simulink model "UAV_Research_Environment"  (R2025a)
settings: Solver=ode23t  StartTime=0.0  StopTime=130  MaxStep=2e-3  RelTol=1e-4  AbsTol=1e-3  EnableMultiTasking=on
InitFcn:
  | skipInitialization = false;
  | 
  | if evalin('base', ...
  |         'exist(''CONTROLLER_TUNING_ACTIVE'',''var'')')
  | 
  |     skipInitialization = evalin('base', ...
  |         'logical(CONTROLLER_TUNING_ACTIVE)');
  | end
  | 
  | if ~skipInitialization
  | 
  |     icraControllerPrepared = false;
  | 
  |     hasICRAVariables = evalin('base', ...
  |         ['exist(''AUTOPILOT'',''var'') && ' ...
  |          'exist(''ICRA_ACTIVE_CONTROLLER'',''var'') && ' ...
  |          'exist(''ICRA_ACTIVE_RUN_ID'',''var'')']);
  | 
  |     if hasICRAVariables
  | 
  |         icraControllerPrepared = evalin('base', ...
  |             ['isstruct(AUTOPILOT) && ' ...
  |              'isfield(AUTOPILOT,''info'') && ' ...
  |              'isfield(AUTOPILOT.info,''ICRAControllerID'') && ' ...
  |              'strcmp(string(AUTOPILOT.info.ICRAControllerID), ' ...
  |                     'string(ICRA_ACTIVE_CONTROLLER))']);
  | 
  |     end
  | 
  |     if icraControllerPrepared
  |         skipInitialization = true;
  |     end
  | end
  | 
  | if ~skipInitialization
  | 
  |     mdl = bdroot;
  | 
  |     mdl_file = get_param(mdl, 'FileName');
  | 
  |     project_root = fileparts(mdl_file);
  | 
  |     init_file = fullfile(project_root, 'initialize_project.m');
  | 
  |     if exist(init_file, 'file')
  | 
  |         run(init_file);
  | 
  |     else
  | 
  |         error('initialize_project.m was not found in the model folder.');
  | 
  |     end
  | end
values from neighbouring files (symbols this model uses):
  A_UAV = struct()    [UAV_analytical.m]
  AUTOPILOT = struct()    [UAV_autopilot.m]
  B_UAV = struct()    [UAV_block.m]
  D = A_UAV.source.propeller_diameter_m    [UAV_analytical.m]    (also in plot_controller_results.m = permute(                  D,                  order); plot_estimator_results.m = permute(              D,              order); plot_mission_results.m = permute(                  D,                  order); plot_touchdown_diagnostics.m = permute(                  D,                  order))
  OPERATOR_MODE = OPERATOR_MODE_MANUAL    [initialize_project.m]    (also in uav_remote_gui.m = uint8(0))
  P_ENV = struct()    [Environment.m]
  P_UAV = struct()    [UAV_simscape.m]
  s = sin(angle)    [uav_remote_gui.m]
  SENSOR = struct()    [UAV_sensors.m]
  TRAJECTORY_CONFIG = struct()    [UAV_trajectories.m]
  TRAJECTORY_ID = uint8(          trajectoryIDNumeric)    [UAV_trajectories.m]
  X = reshape(                  D,                  nt,                  [])    [plot_controller_results.m]    (also in plot_estimator_results.m = reshape(              D,              nt,              []); plot_mission_results.m; plot_touchdown_diagnostics.m; plot_trajectory_3d.m)
  Y = absolutePlanNED(1,:)    [plot_trajectory_3d.m]    (also in uav_remote_gui.m = positionNED(:,1))
  Z = landedCGDown -          absolutePlanNED(3,:)    [plot_trajectory_3d.m]    (also in uav_remote_gui.m = landedCGDown-positionNED(:,3))
undefined symbols (not defined in the file or in its folder): Acceleration_ref, F, fractalcoef, Light, MIL, Position_ref, Velocity_ref, Yaw_ref, YawRate_ref
libraries: sm_lib x49, nesl_utility x29, fl_lib x17, slpidlib x16, simulink x14, ee_lib x5, sdl_lib x4, aerolibwind2 x3, aerolibatmos2 x2, sensorbarometerlib x1, sensorgpslib x1, mspsensorlib x1
(part 3 of 9)

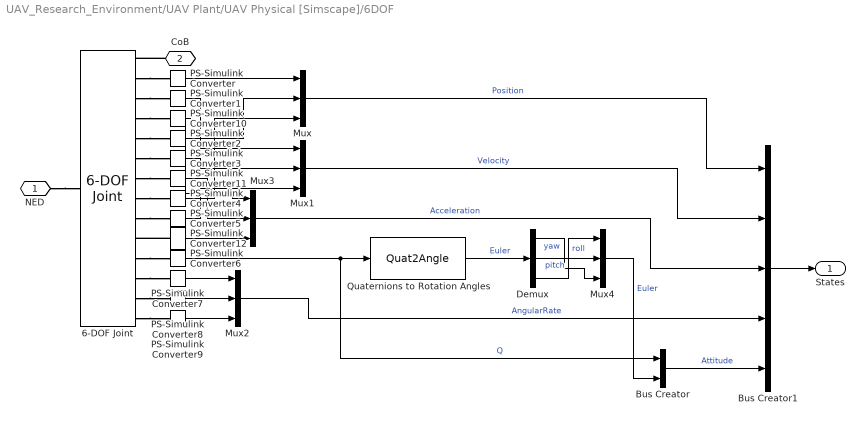
== system UAV_Research_Environment/UAV Plant/UAV Physical [Simscape]/6DOF ==
  6-DOF Joint : sm_lib/Joints/6-DOF Joint  JointMode=Normal  CompositeWrenchDir=FollowerOnBase  CompositeWrenchFrame=BaseFrame  SenseConstraintForce=off  SenseConstraintTorque=off  SenseTotalForce=off  SenseTotalTorque=off  PxPositionTargetSpecify=off  PxPositionTargetPriority=High  PxPositionTargetValue=0  PxPositionTargetValueUnits=m  PxVelocityTargetSpecify=off  PxVelocityTargetPriority=High  PxVelocityTargetValue=0  PxVelocityTargetValueUnits=m/s  PxEquilibriumPosition=0  PxEquilibriumPositionUnits=m  PxSpringStiffness=0  PxSpringStiffnessUnits=N/m  PxDampingCoefficient=0  PxDampingCoefficientUnits=N/(m/s)  PxLowerLimitSpecify=off  PxLowerLimitBound=-1  PxLowerLimitBoundUnits=m  PxLowerLimitStiffness=1e6  PxLowerLimitStiffnessUnits=N/m  PxLowerLimitDamping=1e3  PxLowerLimitDampingUnits=N/(m/s)  PxLowerLimitTransitionRegionWidth=1e-4  PxLowerLimitTransitionRegionWidthUnits=m  PxUpperLimitSpecify=off  PxUpperLimitBound=1  PxUpperLimitBoundUnits=m  PxUpperLimitStiffness=1e6  PxUpperLimitStiffnessUnits=N/m  PxUpperLimitDamping=1e3  PxUpperLimitDampingUnits=N/(m/s)  PxUpperLimitTransitionRegionWidth=1e-4  PxUpperLimitTransitionRegionWidthUnits=m  PxTorqueActuationMode=NoTorque  PxMotionActuationMode=ComputedMotion  PxSensePosition=on  PxSenseVelocity=on  PxSenseAcceleration=on  PxSenseTorqueForce=off  PxSenseLowerLimitTorqueForce=off  PxSenseUpperLimitTorqueForce=off  PyPositionTargetSpecify=off  PyPositionTargetPriority=High  PyPositionTargetValue=0  PyPositionTargetValueUnits=m  PyVelocityTargetSpecify=off  PyVelocityTargetPriority=High  PyVelocityTargetValue=0  PyVelocityTargetValueUnits=m/s  PyEquilibriumPosition=0  PyEquilibriumPositionUnits=m  PySpringStiffness=0  PySpringStiffnessUnits=N/m  PyDampingCoefficient=0  PyDampingCoefficientUnits=N/(m/s)  PyLowerLimitSpecify=off  PyLowerLimitBound=-1  PyLowerLimitBoundUnits=m  PyLowerLimitStiffness=1e6  PyLowerLimitStiffnessUnits=N/m  PyLowerLimitDamping=1e3  PyLowerLimitDampingUnits=N/(m/s)  PyLowerLimitTransitionRegionWidth=1e-4  PyLowerLimitTransitionRegionWidthUnits=m  PyUpperLimitSpecify=off  PyUpperLimitBound=1  PyUpperLimitBoundUnits=m  PyUpperLimitStiffness=1e6  PyUpperLimitStiffnessUnits=N/m  PyUpperLimitDamping=1e3  PyUpperLimitDampingUnits=N/(m/s)  PyUpperLimitTransitionRegionWidth=1e-4  PyUpperLimitTransitionRegionWidthUnits=m  PyTorqueActuationMode=NoTorque  PyMotionActuationMode=ComputedMotion  PySensePosition=on  PySenseVelocity=on  PySenseAcceleration=on  PySenseTorqueForce=off  PySenseLowerLimitTorqueForce=off  PySenseUpperLimitTorqueForce=off  PzPositionTargetSpecify=on  PzPositionTargetPriority=High  PzPositionTargetValue=P_UAV.initial_conditions.position_ned_m(3)  PzPositionTargetValueUnits=m  PzVelocityTargetSpecify=off  PzVelocityTargetPriority=High  PzVelocityTargetValue=0  PzVelocityTargetValueUnits=m/s  PzEquilibriumPosition=0  PzEquilibriumPositionUnits=m  PzSpringStiffness=0  PzSpringStiffnessUnits=N/m  PzDampingCoefficient=0  PzDampingCoefficientUnits=N/(m/s)  PzLowerLimitSpecify=off  PzLowerLimitBound=-1  PzLowerLimitBoundUnits=m  PzLowerLimitStiffness=1e6  PzLowerLimitStiffnessUnits=N/m  PzLowerLimitDamping=1e3  PzLowerLimitDampingUnits=N/(m/s)  PzLowerLimitTransitionRegionWidth=1e-4  PzLowerLimitTransitionRegionWidthUnits=m  PzUpperLimitSpecify=off  PzUpperLimitBound=1  PzUpperLimitBoundUnits=m  PzUpperLimitStiffness=1e6  PzUpperLimitStiffnessUnits=N/m  PzUpperLimitDamping=1e3  PzUpperLimitDampingUnits=N/(m/s)  PzUpperLimitTransitionRegionWidth=1e-4  PzUpperLimitTransitionRegionWidthUnits=m  PzTorqueActuationMode=NoTorque  PzMotionActuationMode=ComputedMotion  PzSensePosition=on  PzSenseVelocity=on  PzSenseAcceleration=on  PzSenseTorqueForce=off  PzSenseLowerLimitTorqueForce=off  PzSenseUpperLimitTorqueForce=off  SphPositionTargetSpecify=off  SphPositionTargetPriority=High  SphPositionTargetRotationMethod=None  SphPositionTargetFollAlignAxisA=+X  SphPositionTargetBaseAlignAxisA=+Y  SphPositionTargetFollAlignAxisB=+Y  SphPositionTargetBaseAlignAxisB=+Z  SphPositionTargetRotationStandardAxis=+Z  SphPositionTargetRotationAngle=0  SphPositionTargetRotationAngleUnits=deg  SphPositionTargetRotationArbitraryAxis=[0 0 1]  SphPositionTargetRotationSequenceAxes=FollowerAxes  SphPositionTargetRotationSequence=XYX  SphPositionTargetRotationSequenceAngles=[0 0 0]  SphPositionTargetRotationSequenceAnglesUnits=deg  SphPositionTargetRotationMatrix=[1 0 0;0 1 0;0 0 1]  SphPositionTargetQuaternion=[1 0 0 0]  SphVelocityTargetSpecify=off  SphVelocityTargetPriority=High  SphVelocityTargetValue=[0 0 0]  SphVelocityTargetValueUnits=deg/s  SphVelocityTargetInFollowerFrame=on  SphEqPosRotationMethod=None  SphEqPosFollAlignAxisA=+X  SphEqPosBaseAlignAxisA=+Y  SphEqPosFollAlignAxisB=+Y  SphEqPosBaseAlignAxisB=+Z  SphEqPosRotationStandardAxis=+Z  SphEqPosRotationAngle=0  SphEqPosRotationAngleUnits=deg  SphEqPosRotationArbitraryAxis=[0 0 1]  SphEqPosRotationSequenceAxes=FollowerAxes  SphEqPosRotationSequence=XYX  SphEqPosRotationSequenceAngles=[0 0 0]  SphEqPosRotationSequenceAnglesUnits=deg  SphEqPosRotationMatrix=[1 0 0;0 1 0;0 0 1]  SphEqPosQuaternion=[1 0 0 0]  SphSpringStiffness=0  SphSpringStiffnessUnits=N*m/deg  SphDampingCoefficient=0  SphDampingCoefficientUnits=N*m/(deg/s)  SphLowerLimitSpecify=off  SphLowerLimitBound=15  SphLowerLimitBoundUnits=deg  SphLowerLimitStiffness=1e4  SphLowerLimitStiffnessUnits=N*m/deg  SphLowerLimitDamping=10  SphLowerLimitDampingUnits=N*m/(deg/s)  SphLowerLimitTransitionRegionWidth=0.1  SphLowerLimitTransitionRegionWidthUnits=deg  SphUpperLimitSpecify=off  SphUpperLimitBound=45  SphUpperLimitBoundUnits=deg  SphUpperLimitStiffness=1e4  SphUpperLimitStiffnessUnits=N*m/deg  SphUpperLimitDamping=10  SphUpperLimitDampingUnits=N*m/(deg/s)  SphUpperLimitTransitionRegionWidth=0.1  SphUpperLimitTransitionRegionWidthUnits=deg  SphTorqueActuationMode=NoTorque  SphActuateTorqueX=off  SphActuateTorqueY=off  SphActuateTorqueZ=off  SphActuateTorque=off  SphActuationFrame=BaseFrame  SphSensePosition=on  SphSenseVelocityX=on  SphSenseVelocityY=on  SphSenseVelocityZ=on  SphSenseVelocity=off  SphSenseAccelerationX=off  SphSenseAccelerationY=off  SphSenseAccelerationZ=off  SphSenseAcceleration=off  SphSenseLowerLimitTorqueMag=off  SphSenseUpperLimitTorqueMag=off  SphSensingFrame=FollowerFrame
  Bus Creator : BusCreator  Inputs=2
  Bus Creator1 : BusCreator  Inputs=5
  Demux : Demux  Outputs=3
  Mux{,1..4} (5 alike) : Mux  Inputs=3
  PS-Simulink Converter{,1..12} (13 alike) : nesl_utility/PS-Simulink Converter  PhysicalDomain=network_engine_domain  SubClassName=ps_output  LeftPortType=input  RightPortType=output  PseudoPeriodic=off  Frequencies=[]  VectorFormat=inherit  Unit=inherit  AffineConversion=off
  Quaternions to Rotation Angles : Quat2Angle
      settings: AttributesFormatString=Rotation Order: %<rotationOrder>
  NED : PMIOPort  Side=Left
  CoB : PMIOPort  Port=2  Side=Right
  States : Outport
  wires:
  PS-Simulink Converter/1 -> Mux/1
  PS-Simulink Converter1/1 -> Mux1/1
  PS-Simulink Converter2/1 -> Mux/2
  PS-Simulink Converter3/1 -> Mux1/2
  PS-Simulink Converter4/1 -> Mux/3
  PS-Simulink Converter5/1 -> Mux1/3
  PS-Simulink Converter6/1 -> Bus Creator/1, Quaternions to Rotation Angles/1  "Q"
  PS-Simulink Converter7/1 -> Mux2/1
  PS-Simulink Converter8/1 -> Mux2/2
  PS-Simulink Converter9/1 -> Mux2/3
  Quaternions to Rotation Angles/1 -> Demux/1  "Euler"
  Mux/1 -> Bus Creator1/1  "Position"
  Mux1/1 -> Bus Creator1/2  "Velocity"
  Mux2/1 -> Bus Creator1/4  "AngularRate"
  Mux3/1 -> Bus Creator1/3  "Acceleration"
  PS-Simulink Converter10/1 -> Mux3/1
  PS-Simulink Converter11/1 -> Mux3/2
  PS-Simulink Converter12/1 -> Mux3/3
  Bus Creator1/1 -> States/1
  Bus Creator/1 -> Bus Creator1/5  "Attitude"
  Demux/1 -> Mux4/3  "yaw"
  Demux/3 -> Mux4/1  "roll"
  Demux/2 -> Mux4/2  "pitch"
  Mux4/1 -> Bus Creator/2  "Euler"
  connections:
  CoB/RConn1 -- 6-DOF Joint/RConn1
  NED/RConn1 -- 6-DOF Joint/LConn1
  6-DOF Joint/RConn2 -- PS-Simulink Converter/LConn1
  6-DOF Joint/RConn3 -- PS-Simulink Converter1/LConn1
  6-DOF Joint/RConn5 -- PS-Simulink Converter2/LConn1
  6-DOF Joint/RConn6 -- PS-Simulink Converter3/LConn1
  6-DOF Joint/RConn8 -- PS-Simulink Converter4/LConn1
  6-DOF Joint/RConn9 -- PS-Simulink Converter5/LConn1
  6-DOF Joint/RConn11 -- PS-Simulink Converter6/LConn1
  6-DOF Joint/RConn12 -- PS-Simulink Converter7/LConn1
  6-DOF Joint/RConn13 -- PS-Simulink Converter8/LConn1
  6-DOF Joint/RConn14 -- PS-Simulink Converter9/LConn1
  6-DOF Joint/RConn4 -- PS-Simulink Converter10/LConn1
  6-DOF Joint/RConn7 -- PS-Simulink Converter11/LConn1
  PS-Simulink Converter12/LConn1 -- 6-DOF Joint/RConn10

== system UAV_Research_Environment/UAV Plant/UAV Physical [Simscape]/Aerodynamics ==
  States : Inport
  Env : Inport  Port=2
  Aerodynamics Forces and Moments : Subsystem
  Demux : Demux  Outputs=6
  "External Force and Torque " : sm_lib/Forces and Torques/External Force and Torque  EnableForceX=on  EnableForceY=on  EnableForceZ=on  EnableForce=off  ForceResolutionFrame=AttachedFrame  EnableTorqueX=on  EnableTorqueY=on  EnableTorqueZ=on  EnableTorque=off  TorqueResolutionFrame=AttachedFrame
  Simulink-PS Converter{,1..5} (6 alike) : nesl_utility/Simulink-PS Converter  PhysicalDomain=network_engine_domain  SubClassName=ps_input  LeftPortType=input  RightPortType=output  PseudoPeriodic=off  Frequencies=[]  NoiseDistribution=none  NoiseParameters=[]  Unit=1  AffineConversion=off  FilteringAndDerivatives=provide  SimscapeFilterOrder=1  InputFilterTimeConstant=0.001  UdotUserProvided=0
  CoB : PMIOPort  Side=Left
  tag scope: Env=global
  wires:
  States/1 -> Aerodynamics Forces and Moments/1(Sim)
  Env/1 -> [Env], Aerodynamics Forces and Moments/2(Env)
  Demux/1 -> Simulink-PS Converter/1
  Demux/2 -> Simulink-PS Converter1/1
  Demux/3 -> Simulink-PS Converter2/1
  Demux/4 -> Simulink-PS Converter3/1
  Demux/5 -> Simulink-PS Converter4/1
  Demux/6 -> Simulink-PS Converter5/1
  Aerodynamics Forces and Moments/1(ForceAndMoment) -> Demux/1
  connections:
  CoB/RConn1 -- "External Force and Torque "/RConn1
  Simulink-PS Converter/RConn1 -- "External Force and Torque "/LConn1
  Simulink-PS Converter1/RConn1 -- "External Force and Torque "/LConn2
  Simulink-PS Converter2/RConn1 -- "External Force and Torque "/LConn3
  Simulink-PS Converter3/RConn1 -- "External Force and Torque "/LConn4
  Simulink-PS Converter4/RConn1 -- "External Force and Torque "/LConn5
  Simulink-PS Converter5/RConn1 -- "External Force and Torque "/LConn6

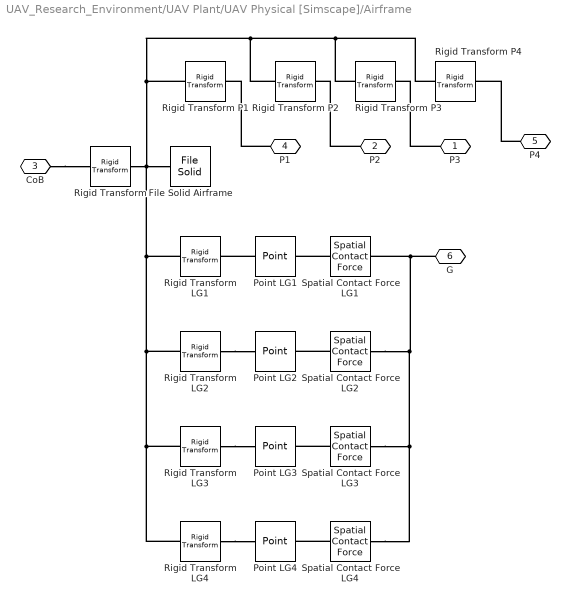
== system UAV_Research_Environment/UAV Plant/UAV Physical [Simscape]/Airframe ==
  File Solid Airframe : sm_lib/Body Elements/File Solid  ExtGeomFileName=CAD/Airframe.step  UnitType=FromFile  ExtGeomFileUnits=m  StepReaderType=HEX  ExportConvexHullGeometry=off  InertiaType=Custom  BasedOnType=Mass  Density=1000  DensityUnits=kg/m^3  Mass=P_UAV.mass.airframe_kg  MassUnits=kg  CenterOfMass=P_UAV.cg.airframe_m  CenterOfMassUnits=m  MomentsOfInertia=P_UAV.inertia.moments_kgm2  MomentsOfInertiaUnits=kg*m^2  ProductsOfInertia=P_UAV.inertia.products_kgm2  ProductsOfInertiaUnits=kg*m^2  GraphicType=FromGeometry  MarkerShape=Sphere  MarkerSize=10  GraphicVisPropType=SimpleVisualProperties  GraphicDiffuseColor=[0.35 0.35 0.35]  GraphicOpacity=1  GraphicSpecularColor=[0.5 0.5 0.5 1.0]  GraphicAmbientColor=[0.15 0.15 0.15 1.0]  GraphicEmissiveColor=[0.0 0.0 0.0 1.0]  GraphicShininess=75  DoExposeReferenceFrame=on  SerializedFrames=<Frames/>
  Point LG{1..4} (4 alike) : sm_lib/Curves and Surfaces/Point  GraphicType=None  MarkerShape=Sphere  MarkerSize=10  GraphicVisPropType=SimpleVisualProperties  GraphicDiffuseColor=[0.5 0.5 0.5]  GraphicOpacity=1  GraphicSpecularColor=[0.5 0.5 0.5 1.0]  GraphicAmbientColor=[0.15 0.15 0.15 1.0]  GraphicEmissiveColor=[0.0 0.0 0.0 1.0]  GraphicShininess=75
  Rigid Transform : sm_lib/Frames and Transforms/Rigid Transform  RotationMethod=AlignedAxes  FollAlignAxisA=+Z  BaseAlignAxisA=+X  FollAlignAxisB=+X  BaseAlignAxisB=-Y  RotationStandardAxis=+Z  RotationAngle=0  RotationAngleUnits=deg  RotationArbitraryAxis=[0 0 1]  RotationSequenceAxes=FollowerAxes  RotationSequence=XYX  RotationSequenceAngles=[0 0 0]  RotationSequenceAnglesUnits=deg  RotationMatrix=[1 0 0;0 1 0;0 0 1]  Quaternion=[1 0 0 0]  TranslationMethod=Cartesian  TranslationCartesianOffset=-P_UAV.cg.airframe_body_m.'  TranslationCartesianOffsetUnits=m  TranslationStandardAxis=+Z  TranslationStandardOffset=0  TranslationStandardOffsetUnits=m  TranslationROffset=0  TranslationROffsetUnits=m  TranslationThetaOffset=0  TranslationThetaOffsetUnits=deg  TranslationZOffset=0  TranslationZOffsetUnits=m
  Rigid Transform LG1 : sm_lib/Frames and Transforms/Rigid Transform  RotationMethod=None  FollAlignAxisA=+Z  BaseAlignAxisA=+X  FollAlignAxisB=+X  BaseAlignAxisB=-Y  RotationStandardAxis=+Z  RotationAngle=0  RotationAngleUnits=deg  RotationArbitraryAxis=[0 0 1]  RotationSequenceAxes=FollowerAxes  RotationSequence=XYX  RotationSequenceAngles=[0 0 0]  RotationSequenceAnglesUnits=deg  RotationMatrix=[1 0 0;0 1 0;0 0 1]  Quaternion=[1 0 0 0]  TranslationMethod=Cartesian  TranslationCartesianOffset=P_UAV.contact.point1_cad_m  TranslationCartesianOffsetUnits=m  TranslationStandardAxis=+Z  TranslationStandardOffset=0  TranslationStandardOffsetUnits=m  TranslationROffset=0  TranslationROffsetUnits=m  TranslationThetaOffset=0  TranslationThetaOffsetUnits=deg  TranslationZOffset=0  TranslationZOffsetUnits=m
  Rigid Transform LG2 : sm_lib/Frames and Transforms/Rigid Transform  RotationMethod=None  FollAlignAxisA=+Z  BaseAlignAxisA=+X  FollAlignAxisB=+X  BaseAlignAxisB=-Y  RotationStandardAxis=+Z  RotationAngle=0  RotationAngleUnits=deg  RotationArbitraryAxis=[0 0 1]  RotationSequenceAxes=FollowerAxes  RotationSequence=XYX  RotationSequenceAngles=[0 0 0]  RotationSequenceAnglesUnits=deg  RotationMatrix=[1 0 0;0 1 0;0 0 1]  Quaternion=[1 0 0 0]  TranslationMethod=Cartesian  TranslationCartesianOffset=P_UAV.contact.point2_cad_m  TranslationCartesianOffsetUnits=m  TranslationStandardAxis=+Z  TranslationStandardOffset=0  TranslationStandardOffsetUnits=m  TranslationROffset=0  TranslationROffsetUnits=m  TranslationThetaOffset=0  TranslationThetaOffsetUnits=deg  TranslationZOffset=0  TranslationZOffsetUnits=m
  Rigid Transform LG3 : sm_lib/Frames and Transforms/Rigid Transform  RotationMethod=None  FollAlignAxisA=+Z  BaseAlignAxisA=+X  FollAlignAxisB=+X  BaseAlignAxisB=-Y  RotationStandardAxis=+Z  RotationAngle=0  RotationAngleUnits=deg  RotationArbitraryAxis=[0 0 1]  RotationSequenceAxes=FollowerAxes  RotationSequence=XYX  RotationSequenceAngles=[0 0 0]  RotationSequenceAnglesUnits=deg  RotationMatrix=[1 0 0;0 1 0;0 0 1]  Quaternion=[1 0 0 0]  TranslationMethod=Cartesian  TranslationCartesianOffset=P_UAV.contact.point3_cad_m  TranslationCartesianOffsetUnits=m  TranslationStandardAxis=+Z  TranslationStandardOffset=0  TranslationStandardOffsetUnits=m  TranslationROffset=0  TranslationROffsetUnits=m  TranslationThetaOffset=0  TranslationThetaOffsetUnits=deg  TranslationZOffset=0  TranslationZOffsetUnits=m
  Rigid Transform LG4 : sm_lib/Frames and Transforms/Rigid Transform  RotationMethod=None  FollAlignAxisA=+Z  BaseAlignAxisA=+X  FollAlignAxisB=+X  BaseAlignAxisB=-Y  RotationStandardAxis=+Z  RotationAngle=0  RotationAngleUnits=deg  RotationArbitraryAxis=[0 0 1]  RotationSequenceAxes=FollowerAxes  RotationSequence=XYX  RotationSequenceAngles=[0 0 0]  RotationSequenceAnglesUnits=deg  RotationMatrix=[1 0 0;0 1 0;0 0 1]  Quaternion=[1 0 0 0]  TranslationMethod=Cartesian  TranslationCartesianOffset=P_UAV.contact.point4_cad_m  TranslationCartesianOffsetUnits=m  TranslationStandardAxis=+Z  TranslationStandardOffset=0  TranslationStandardOffsetUnits=m  TranslationROffset=0  TranslationROffsetUnits=m  TranslationThetaOffset=0  TranslationThetaOffsetUnits=deg  TranslationZOffset=0  TranslationZOffsetUnits=m
  Rigid Transform P1 : sm_lib/Frames and Transforms/Rigid Transform  RotationMethod=AlignedAxes  FollAlignAxisA=+Z  BaseAlignAxisA=+Y  FollAlignAxisB=+X  BaseAlignAxisB=+Z  RotationStandardAxis=+Z  RotationAngle=0  RotationAngleUnits=deg  RotationArbitraryAxis=[0 0 1]  RotationSequenceAxes=FollowerAxes  RotationSequence=XYX  RotationSequenceAngles=[0 0 0]  RotationSequenceAnglesUnits=deg  RotationMatrix=[1 0 0;0 1 0;0 0 1]  Quaternion=[1 0 0 0]  TranslationMethod=Cartesian  TranslationCartesianOffset=P_UAV.motor.position1_cad_m  TranslationCartesianOffsetUnits=m  TranslationStandardAxis=+Z  TranslationStandardOffset=0  TranslationStandardOffsetUnits=m  TranslationROffset=0  TranslationROffsetUnits=m  TranslationThetaOffset=0  TranslationThetaOffsetUnits=deg  TranslationZOffset=0  TranslationZOffsetUnits=m
  Rigid Transform P2 : sm_lib/Frames and Transforms/Rigid Transform  RotationMethod=AlignedAxes  FollAlignAxisA=+Z  BaseAlignAxisA=+Y  FollAlignAxisB=+X  BaseAlignAxisB=+Z  RotationStandardAxis=+Z  RotationAngle=0  RotationAngleUnits=deg  RotationArbitraryAxis=[0 0 1]  RotationSequenceAxes=FollowerAxes  RotationSequence=XYX  RotationSequenceAngles=[0 0 0]  RotationSequenceAnglesUnits=deg  RotationMatrix=[1 0 0;0 1 0;0 0 1]  Quaternion=[1 0 0 0]  TranslationMethod=Cartesian  TranslationCartesianOffset=P_UAV.motor.position2_cad_m  TranslationCartesianOffsetUnits=m  TranslationStandardAxis=+Z  TranslationStandardOffset=0  TranslationStandardOffsetUnits=m  TranslationROffset=0  TranslationROffsetUnits=m  TranslationThetaOffset=0  TranslationThetaOffsetUnits=deg  TranslationZOffset=0  TranslationZOffsetUnits=m
  Rigid Transform P3 : sm_lib/Frames and Transforms/Rigid Transform  RotationMethod=AlignedAxes  FollAlignAxisA=+Z  BaseAlignAxisA=+Y  FollAlignAxisB=+X  BaseAlignAxisB=+Z  RotationStandardAxis=+Z  RotationAngle=0  RotationAngleUnits=deg  RotationArbitraryAxis=[0 0 1]  RotationSequenceAxes=FollowerAxes  RotationSequence=XYX  RotationSequenceAngles=[0 0 0]  RotationSequenceAnglesUnits=deg  RotationMatrix=[1 0 0;0 1 0;0 0 1]  Quaternion=[1 0 0 0]  TranslationMethod=Cartesian  TranslationCartesianOffset=P_UAV.motor.position3_cad_m  TranslationCartesianOffsetUnits=m  TranslationStandardAxis=+Z  TranslationStandardOffset=0  TranslationStandardOffsetUnits=m  TranslationROffset=0  TranslationROffsetUnits=m  TranslationThetaOffset=0  TranslationThetaOffsetUnits=deg  TranslationZOffset=0  TranslationZOffsetUnits=m
  Rigid Transform P4 : sm_lib/Frames and Transforms/Rigid Transform  RotationMethod=AlignedAxes  FollAlignAxisA=+Z  BaseAlignAxisA=+Y  FollAlignAxisB=+X  BaseAlignAxisB=+Z  RotationStandardAxis=+Z  RotationAngle=0  RotationAngleUnits=deg  RotationArbitraryAxis=[0 0 1]  RotationSequenceAxes=FollowerAxes  RotationSequence=XYX  RotationSequenceAngles=[0 0 0]  RotationSequenceAnglesUnits=deg  RotationMatrix=[1 0 0;0 1 0;0 0 1]  Quaternion=[1 0 0 0]  TranslationMethod=Cartesian  TranslationCartesianOffset=P_UAV.motor.position4_cad_m  TranslationCartesianOffsetUnits=m  TranslationStandardAxis=+Z  TranslationStandardOffset=0  TranslationStandardOffsetUnits=m  TranslationROffset=0  TranslationROffsetUnits=m  TranslationThetaOffset=0  TranslationThetaOffsetUnits=deg  TranslationZOffset=0  TranslationZOffsetUnits=m
  Spatial Contact Force LG{1..4} (4 alike) : sm_lib/Forces and Torques/Spatial Contact Force  SenseSeparationDistance=off  NormalForceType=SmoothSpringDamper  NormalStiffness=P_ENV.ground.contact.stiffness_N_m  NormalStiffnessUnits=N/m  NormalDamping=P_ENV.ground.contact.damping_N_s_m  NormalDampingUnits=N/(m/s)  NormalTransitionRegionWidth=P_ENV.ground.contact.transition_width_m  NormalTransitionRegionWidthUnits=m  FrictionType=SmoothStickSlip  CoefficientOfStaticFriction=P_ENV.ground.contact.static_friction  CoefficientOfDynamicFriction=P_ENV.ground.contact.dynamic_friction  FrictionalCriticalVelocity=P_ENV.ground.contact.critical_velocity_m_s  FrictionalCriticalVelocityUnits=m/s  SenseContactSignal=off  SensePenetrationDepth=off  SenseNormalVelocity=off  SenseTangentialVelocity=off  SensingForceTorqueDirection=BaseOnFollower  SensingForceTorqueResolutionFrame=ContactFrame  SenseNormalForce=off  SenseNormalForceMagnitude=off  SenseNormalTorque=off  SenseFrictionalForce=off  SenseFrictionalForceMagnitude=off  SenseFrictionalTorque=off  SenseTotalForce=off  SenseTotalTorque=off  SenseContactBaseRotation=off  SenseContactBaseTranslation=off  SenseContactFollowerRotation=off  SenseContactFollowerTranslation=off  ZeroCrossDetectContactStartAndEnd=on
  P3 : PMIOPort  Side=Left
  P2 : PMIOPort  Port=2  Side=Left
  CoB : PMIOPort  Port=3  Side=Left
  P1 : PMIOPort  Port=4  Side=Right
  P4 : PMIOPort  Port=5  Side=Right
  G : PMIOPort  Port=6  Side=Right
  connections:
  Rigid Transform LG4/LConn1 -- File Solid Airframe/RConn1 -- Rigid Transform/RConn1 -- Rigid Transform P2/LConn1 -- Rigid Transform P4/LConn1 -- Rigid Transform P3/LConn1 -- Rigid Transform P1/LConn1 -- Rigid Transform LG1/LConn1 -- Rigid Transform LG2/LConn1 -- Rigid Transform LG3/LConn1
  CoB/RConn1 -- Rigid Transform/LConn1
  P1/RConn1 -- Rigid Transform P1/RConn1
  P2/RConn1 -- Rigid Transform P2/RConn1
  P3/RConn1 -- Rigid Transform P3/RConn1
  P4/RConn1 -- Rigid Transform P4/RConn1
  Spatial Contact Force LG3/RConn1 -- Spatial Contact Force LG1/RConn1 -- G/RConn1 -- Spatial Contact Force LG2/RConn1 -- Spatial Contact Force LG4/RConn1
  Rigid Transform LG2/RConn1 -- Point LG2/LConn1
  Rigid Transform LG4/RConn1 -- Point LG4/LConn1
  Rigid Transform LG3/RConn1 -- Point LG3/LConn1
  Spatial Contact Force LG3/LConn1 -- Point LG3/RConn1
  Spatial Contact Force LG1/LConn1 -- Point LG1/RConn1
  Point LG1/LConn1 -- Rigid Transform LG1/RConn1
  Spatial Contact Force LG4/LConn1 -- Point LG4/RConn1
  Spatial Contact Force LG2/LConn1 -- Point LG2/RConn1

== system UAV_Research_Environment/UAV Plant/UAV Physical [Simscape]/Battery ==
  Connection Label3 : ConnectionLabel  Label=VCC
  Connection Label4 : ConnectionLabel  Label=GND
  DC Voltage Source : ee_lib/Additional Components/SPICE Sources/DC Voltage Source  DC=P_UAV.battery.ideal_voltage_V V
  Electrical Reference : fl_lib/Electrical/Electrical Elements/Electrical Reference
  VCC : PMIOPort  Side=Left
  GND : PMIOPort  Port=2  Side=Left
  connections:
  Connection Label3/LConn1 -- VCC/RConn1 -- DC Voltage Source/LConn1
  Connection Label4/LConn1 -- GND/RConn1 -- Electrical Reference/LConn1 -- DC Voltage Source/RConn1

== system UAV_Research_Environment/UAV Plant/UAV Physical [Simscape]/Ground ==
  "Infinite Plane " : sm_lib/Curves and Surfaces/Infinite Plane  GraphicType=Rectangle  GraphicPlaneWidth=10  GraphicPlaneWidthUnits=m  GraphicPlaneHeight=10  GraphicPlaneHeightUnits=m  GraphicVisPropType=SimpleVisualProperties  GraphicDiffuseColor=[0.902 0.902 0.902]  GraphicOpacity=1  GraphicSpecularColor=[0.5 0.5 0.5 1.0]  GraphicAmbientColor=[0.15 0.15 0.15 1.0]  GraphicEmissiveColor=[0.0 0.0 0.0 1.0]  GraphicShininess=75
  "Rigid Transform " : sm_lib/Frames and Transforms/Rigid Transform  RotationMethod=RotationSequence  FollAlignAxisA=+X  BaseAlignAxisA=+Y  FollAlignAxisB=+Y  BaseAlignAxisB=+Z  RotationStandardAxis=+Z  RotationAngle=0  RotationAngleUnits=deg  RotationArbitraryAxis=[0 0 1]  RotationSequenceAxes=FollowerAxes  RotationSequence=XYZ  RotationSequenceAngles=[180 0 0]  RotationSequenceAnglesUnits=deg  RotationMatrix=[1 0 0;0 1 0;0 0 1]  Quaternion=[1 0 0 0]  TranslationMethod=None  TranslationCartesianOffset=[0 0 0]  TranslationCartesianOffsetUnits=m  TranslationStandardAxis=+Z  TranslationStandardOffset=0  TranslationStandardOffsetUnits=m  TranslationROffset=0  TranslationROffsetUnits=m  TranslationThetaOffset=0  TranslationThetaOffsetUnits=deg  TranslationZOffset=0  TranslationZOffsetUnits=m
  NED : PMIOPort  Side=Left
  G : PMIOPort  Port=2  Side=Left
  connections:
  "Infinite Plane "/LConn1 -- "Rigid Transform "/RConn1
  G/RConn1 -- "Infinite Plane "/RConn1
  NED/RConn1 -- "Rigid Transform "/LConn1

== system UAV_Research_Environment/UAV Plant/UAV Physical [Simscape]/Motor ESC 1 ==
  wCmd : Inport
  Mechanical Rotational Reference1 : fl_lib/Mechanical/Rotational Elements/Mechanical Rotational Reference
  Mechanical Rotational Reference : fl_lib/Mechanical/Rotational Elements/Mechanical Rotational Reference
  "Motor & Drive (System Level) " : ee_lib/Electromechanical/Motor & Drive (System Level)  torque_speed_param=ee.enum.electromech.envelope.torque_power  overtorque_param=ee.enum.electromech.overtorque.no  T_t=[.09, .08, .07, 0] N*m  T_t_intermittent=[.36, .32, .28, 0] N*m  T_t_2D=[.09, .09, .09; .08, .08, .08; .07, .07, .07; 0, 0, 0] N*m  T_t_intermittent_2D=[.36, .36, .36; .32, .32, .32; .28, .28, .28; 0, 0, 0] N*m  w_t=[0, 3750, 7500, 8000] rpm  vdc_t=[6, 12, 24] V  torque_max="P_UAV.drive.max_torque_Nm  N*m"  power_max="P_UAV.drive.max_power_W  W"  torque_max_intermittent=0.4 N*m  power_max_intermittent=120 W  time_overtorque=30 s  time_recover=60 s  Tc="P_UAV.drive.torque_control_time_constant_s  s"  EnableSwitch=false  losses_param=1  eff=P_UAV.drive.efficiency_percent  w_eff="P_UAV.drive.efficiency_speed_rpm  rpm"  T_eff="P_UAV.drive.efficiency_torque_Nm  N*m"  Piron="P_UAV.drive.iron_loss_W  W"  Pbase="P_UAV.drive.fixed_loss_W  W"  w_eff_vec=[-8000, -4000, 0, 4000, 8000] rpm  T_eff_vec=[0, .03, .06, .09] N*m  v_eff_vec=[100, 250, 400] V  losses_mat=[1.49, 1.67, 2.21, 3.1; .42, .69, 1.14, 2.03; .06, .24, .78, 1.68; .42, .69, 1.14, 2.03; 1.49, 1.67, 2.21, 3.1] W  efficiency_mat=[95, 95, 95, 95; 95, 95, 95, 95; 95, 95, 95, 95; 95, 95, 95, 95; 95, 95, 95, 95]  losses_mat_3D=ones(5, 4, 3) W  efficiency_mat_3D=95 * ones(5, 4, 3)  Res=P_UAV.drive.external_supply_resistance_Ohm Ohm  J="P_UAV.drive.rotor_inertia_kgm2  kg*m^2"  lam="P_UAV.drive.rotor_damping_Nm_s_rad  N*m*s/rad"  speed0=P_UAV.drive.initial_speed_rpm rpm  faulted_specify=off  faulted_priority=None  faulted=0  faulted_nominal_specify=off  faulted_nominal_value=1  faulted_nominal_unit=1  isSwitchedOff_specify=off  isSwitchedOff_priority=None  isSwitchedOff=0  isSwitchedOff_nominal_specify=off  isSwitchedOff_nominal_value=1  isSwitchedOff_nominal_unit=1  torqueLimitContinuous_specify=off  torqueLimitContinuous_priority=None  torqueLimitContinuous=0 N*m  torqueLimitContinuous_nominal_specify=off  torqueLimitContinuous_nominal_value=1  torqueLimitContinuous_nominal_unit=N*m  alpha=3.93e-3 1/K  Tmeas=25 degC  Tmeas2=125 degC  losses_mat_T2=[1.49, 1.74, 2.49, 3.74; .42, .67, 1.42, 2.67; .06, .31, 1.06, 2.31; .42, .67, 1.42, 2.67; 1.49, 1.74, 2.49, 3.74] W  efficiency_mat_T2=[95, 95, 95, 95; 95, 95, 95, 95; 95, 95, 95, 95; 95, 95, 95, 95; 95, 95, 95, 95]  losses_mat_3D_T2=ones(5, 4, 3) W  efficiency_mat_3D_T2=95 * ones(5, 4, 3)  thermal_mass=100 J/K  initial_temperature=25 degC
  PS-Simulink Converter : nesl_utility/PS-Simulink Converter  PhysicalDomain=network_engine_domain  SubClassName=ps_output  LeftPortType=input  RightPortType=output  PseudoPeriodic=off  Frequencies=[]  VectorFormat=inherit  Unit=inherit  AffineConversion=off
  "Rotational Multibody Interface " : fl_lib/Mechanical/Multibody Interfaces/Rotational Multibody Interface
  Simulink-PS Converter : nesl_utility/Simulink-PS Converter  PhysicalDomain=network_engine_domain  SubClassName=ps_input  LeftPortType=input  RightPortType=output  PseudoPeriodic=off  Frequencies=[]  NoiseDistribution=none  NoiseParameters=[]  Unit=1  AffineConversion=off  FilteringAndDerivatives=filter  SimscapeFilterOrder=1  InputFilterTimeConstant=0.001  UdotUserProvided=0
  Speed PI Control : Subsystem
  Torque : PMIOPort  Side=Left
  w : PMIOPort  Port=2  Side=Left
  GND : PMIOPort  Port=3  Side=Left
  VCC : PMIOPort  Port=4  Side=Left
  wires:
  PS-Simulink Converter/1 -> Speed PI Control/2(w)
  wCmd/1 -> Speed PI Control/1(wCmd)
  Speed PI Control/1(TorqueCmd) -> Simulink-PS Converter/1
  connections:
  VCC/RConn1 -- "Motor & Drive (System Level) "/LConn1
  "Rotational Multibody Interface "/LConn2 -- Mechanical Rotational Reference/LConn1
  "Rotational Multibody Interface "/RConn2 -- "Motor & Drive (System Level) "/LConn3
  Mechanical Rotational Reference1/LConn1 -- "Motor & Drive (System Level) "/RConn3
  "Motor & Drive (System Level) "/RConn1 -- GND/RConn1
  PS-Simulink Converter/LConn1 -- "Motor & Drive (System Level) "/RConn2
  Simulink-PS Converter/RConn1 -- "Motor & Drive (System Level) "/LConn2
  w/RConn1 -- "Rotational Multibody Interface "/RConn1
  Torque/RConn1 -- "Rotational Multibody Interface "/LConn1

== system UAV_Research_Environment/UAV Plant/UAV Physical [Simscape]/Motor ESC 2 ==
  wCmd : Inport
  Mechanical Rotational Reference1 : fl_lib/Mechanical/Rotational Elements/Mechanical Rotational Reference
  Mechanical Rotational Reference : fl_lib/Mechanical/Rotational Elements/Mechanical Rotational Reference
  "Motor & Drive (System Level) " : ee_lib/Electromechanical/Motor & Drive (System Level)  torque_speed_param=ee.enum.electromech.envelope.torque_power  overtorque_param=ee.enum.electromech.overtorque.no  T_t=[.09, .08, .07, 0] N*m  T_t_intermittent=[.36, .32, .28, 0] N*m  T_t_2D=[.09, .09, .09; .08, .08, .08; .07, .07, .07; 0, 0, 0] N*m  T_t_intermittent_2D=[.36, .36, .36; .32, .32, .32; .28, .28, .28; 0, 0, 0] N*m  w_t=[0, 3750, 7500, 8000] rpm  vdc_t=[6, 12, 24] V  torque_max="P_UAV.drive.max_torque_Nm  N*m"  power_max="P_UAV.drive.max_power_W  W"  torque_max_intermittent=0.4 N*m  power_max_intermittent=120 W  time_overtorque=30 s  time_recover=60 s  Tc="P_UAV.drive.torque_control_time_constant_s  s"  EnableSwitch=false  losses_param=1  eff=P_UAV.drive.efficiency_percent  w_eff="P_UAV.drive.efficiency_speed_rpm  rpm"  T_eff="P_UAV.drive.efficiency_torque_Nm  N*m"  Piron="P_UAV.drive.iron_loss_W  W"  Pbase="P_UAV.drive.fixed_loss_W  W"  w_eff_vec=[-8000, -4000, 0, 4000, 8000] rpm  T_eff_vec=[0, .03, .06, .09] N*m  v_eff_vec=[100, 250, 400] V  losses_mat=[1.49, 1.67, 2.21, 3.1; .42, .69, 1.14, 2.03; .06, .24, .78, 1.68; .42, .69, 1.14, 2.03; 1.49, 1.67, 2.21, 3.1] W  efficiency_mat=[95, 95, 95, 95; 95, 95, 95, 95; 95, 95, 95, 95; 95, 95, 95, 95; 95, 95, 95, 95]  losses_mat_3D=ones(5, 4, 3) W  efficiency_mat_3D=95 * ones(5, 4, 3)  Res=P_UAV.drive.external_supply_resistance_Ohm Ohm  J="P_UAV.drive.rotor_inertia_kgm2  kg*m^2"  lam="P_UAV.drive.rotor_damping_Nm_s_rad  N*m*s/rad"  speed0=P_UAV.drive.initial_speed_rpm rpm  faulted_specify=off  faulted_priority=None  faulted=0  faulted_nominal_specify=off  faulted_nominal_value=1  faulted_nominal_unit=1  isSwitchedOff_specify=off  isSwitchedOff_priority=None  isSwitchedOff=0  isSwitchedOff_nominal_specify=off  isSwitchedOff_nominal_value=1  isSwitchedOff_nominal_unit=1  torqueLimitContinuous_specify=off  torqueLimitContinuous_priority=None  torqueLimitContinuous=0 N*m  torqueLimitContinuous_nominal_specify=off  torqueLimitContinuous_nominal_value=1  torqueLimitContinuous_nominal_unit=N*m  alpha=3.93e-3 1/K  Tmeas=25 degC  Tmeas2=125 degC  losses_mat_T2=[1.49, 1.74, 2.49, 3.74; .42, .67, 1.42, 2.67; .06, .31, 1.06, 2.31; .42, .67, 1.42, 2.67; 1.49, 1.74, 2.49, 3.74] W  efficiency_mat_T2=[95, 95, 95, 95; 95, 95, 95, 95; 95, 95, 95, 95; 95, 95, 95, 95; 95, 95, 95, 95]  losses_mat_3D_T2=ones(5, 4, 3) W  efficiency_mat_3D_T2=95 * ones(5, 4, 3)  thermal_mass=100 J/K  initial_temperature=25 degC
  PS-Simulink Converter : nesl_utility/PS-Simulink Converter  PhysicalDomain=network_engine_domain  SubClassName=ps_output  LeftPortType=input  RightPortType=output  PseudoPeriodic=off  Frequencies=[]  VectorFormat=inherit  Unit=inherit  AffineConversion=off
  "Rotational Multibody Interface " : fl_lib/Mechanical/Multibody Interfaces/Rotational Multibody Interface
  Simulink-PS Converter : nesl_utility/Simulink-PS Converter  PhysicalDomain=network_engine_domain  SubClassName=ps_input  LeftPortType=input  RightPortType=output  PseudoPeriodic=off  Frequencies=[]  NoiseDistribution=none  NoiseParameters=[]  Unit=1  AffineConversion=off  FilteringAndDerivatives=filter  SimscapeFilterOrder=1  InputFilterTimeConstant=0.001  UdotUserProvided=0
  Speed PI Control : Subsystem
  Torque : PMIOPort  Side=Left
  w : PMIOPort  Port=2  Side=Left
  VCC : PMIOPort  Port=3  Side=Right
  GND : PMIOPort  Port=4  Side=Right
  wires:
  PS-Simulink Converter/1 -> Speed PI Control/2(w)
  wCmd/1 -> Speed PI Control/1(wCmd)
  Speed PI Control/1(TorqueCmd) -> Simulink-PS Converter/1
  connections:
  VCC/RConn1 -- "Motor & Drive (System Level) "/LConn1
  "Rotational Multibody Interface "/LConn2 -- Mechanical Rotational Reference/LConn1
  "Rotational Multibody Interface "/RConn2 -- "Motor & Drive (System Level) "/LConn3
  Mechanical Rotational Reference1/LConn1 -- "Motor & Drive (System Level) "/RConn3
  "Motor & Drive (System Level) "/RConn1 -- GND/RConn1
  PS-Simulink Converter/LConn1 -- "Motor & Drive (System Level) "/RConn2
  Simulink-PS Converter/RConn1 -- "Motor & Drive (System Level) "/LConn2
  w/RConn1 -- "Rotational Multibody Interface "/RConn1
  Torque/RConn1 -- "Rotational Multibody Interface "/LConn1

== system UAV_Research_Environment/UAV Plant/UAV Physical [Simscape]/Motor ESC 3 ==
  wCmd : Inport
  Mechanical Rotational Reference1 : fl_lib/Mechanical/Rotational Elements/Mechanical Rotational Reference
  Mechanical Rotational Reference : fl_lib/Mechanical/Rotational Elements/Mechanical Rotational Reference
  "Motor & Drive (System Level) " : ee_lib/Electromechanical/Motor & Drive (System Level)  torque_speed_param=ee.enum.electromech.envelope.torque_power  overtorque_param=ee.enum.electromech.overtorque.no  T_t=[.09, .08, .07, 0] N*m  T_t_intermittent=[.36, .32, .28, 0] N*m  T_t_2D=[.09, .09, .09; .08, .08, .08; .07, .07, .07; 0, 0, 0] N*m  T_t_intermittent_2D=[.36, .36, .36; .32, .32, .32; .28, .28, .28; 0, 0, 0] N*m  w_t=[0, 3750, 7500, 8000] rpm  vdc_t=[6, 12, 24] V  torque_max="P_UAV.drive.max_torque_Nm  N*m"  power_max="P_UAV.drive.max_power_W  W"  torque_max_intermittent=0.4 N*m  power_max_intermittent=120 W  time_overtorque=30 s  time_recover=60 s  Tc="P_UAV.drive.torque_control_time_constant_s  s"  EnableSwitch=false  losses_param=1  eff=P_UAV.drive.efficiency_percent  w_eff="P_UAV.drive.efficiency_speed_rpm  rpm"  T_eff="P_UAV.drive.efficiency_torque_Nm  N*m"  Piron="P_UAV.drive.iron_loss_W  W"  Pbase="P_UAV.drive.fixed_loss_W  W"  w_eff_vec=[-8000, -4000, 0, 4000, 8000] rpm  T_eff_vec=[0, .03, .06, .09] N*m  v_eff_vec=[100, 250, 400] V  losses_mat=[1.49, 1.67, 2.21, 3.1; .42, .69, 1.14, 2.03; .06, .24, .78, 1.68; .42, .69, 1.14, 2.03; 1.49, 1.67, 2.21, 3.1] W  efficiency_mat=[95, 95, 95, 95; 95, 95, 95, 95; 95, 95, 95, 95; 95, 95, 95, 95; 95, 95, 95, 95]  losses_mat_3D=ones(5, 4, 3) W  efficiency_mat_3D=95 * ones(5, 4, 3)  Res=P_UAV.drive.external_supply_resistance_Ohm Ohm  J="P_UAV.drive.rotor_inertia_kgm2  kg*m^2"  lam="P_UAV.drive.rotor_damping_Nm_s_rad  N*m*s/rad"  speed0=P_UAV.drive.initial_speed_rpm rpm  faulted_specify=off  faulted_priority=None  faulted=0  faulted_nominal_specify=off  faulted_nominal_value=1  faulted_nominal_unit=1  isSwitchedOff_specify=off  isSwitchedOff_priority=None  isSwitchedOff=0  isSwitchedOff_nominal_specify=off  isSwitchedOff_nominal_value=1  isSwitchedOff_nominal_unit=1  torqueLimitContinuous_specify=off  torqueLimitContinuous_priority=None  torqueLimitContinuous=0 N*m  torqueLimitContinuous_nominal_specify=off  torqueLimitContinuous_nominal_value=1  torqueLimitContinuous_nominal_unit=N*m  alpha=3.93e-3 1/K  Tmeas=25 degC  Tmeas2=125 degC  losses_mat_T2=[1.49, 1.74, 2.49, 3.74; .42, .67, 1.42, 2.67; .06, .31, 1.06, 2.31; .42, .67, 1.42, 2.67; 1.49, 1.74, 2.49, 3.74] W  efficiency_mat_T2=[95, 95, 95, 95; 95, 95, 95, 95; 95, 95, 95, 95; 95, 95, 95, 95; 95, 95, 95, 95]  losses_mat_3D_T2=ones(5, 4, 3) W  efficiency_mat_3D_T2=95 * ones(5, 4, 3)  thermal_mass=100 J/K  initial_temperature=25 degC
  PS-Simulink Converter : nesl_utility/PS-Simulink Converter  PhysicalDomain=network_engine_domain  SubClassName=ps_output  LeftPortType=input  RightPortType=output  PseudoPeriodic=off  Frequencies=[]  VectorFormat=inherit  Unit=inherit  AffineConversion=off
  "Rotational Multibody Interface " : fl_lib/Mechanical/Multibody Interfaces/Rotational Multibody Interface
  Simulink-PS Converter : nesl_utility/Simulink-PS Converter  PhysicalDomain=network_engine_domain  SubClassName=ps_input  LeftPortType=input  RightPortType=output  PseudoPeriodic=off  Frequencies=[]  NoiseDistribution=none  NoiseParameters=[]  Unit=1  AffineConversion=off  FilteringAndDerivatives=filter  SimscapeFilterOrder=1  InputFilterTimeConstant=0.001  UdotUserProvided=0
  Speed PI Control : Subsystem
  Torque : PMIOPort  Side=Left
  w : PMIOPort  Port=2  Side=Left
  VCC : PMIOPort  Port=3  Side=Left
  GND : PMIOPort  Port=4  Side=Left
  wires:
  PS-Simulink Converter/1 -> Speed PI Control/2(w)
  wCmd/1 -> Speed PI Control/1(wCmd)
  Speed PI Control/1(TorqueCmd) -> Simulink-PS Converter/1
  connections:
  VCC/RConn1 -- "Motor & Drive (System Level) "/LConn1
  "Rotational Multibody Interface "/LConn2 -- Mechanical Rotational Reference/LConn1
  "Rotational Multibody Interface "/RConn2 -- "Motor & Drive (System Level) "/LConn3
  Mechanical Rotational Reference1/LConn1 -- "Motor & Drive (System Level) "/RConn3
  "Motor & Drive (System Level) "/RConn1 -- GND/RConn1
  PS-Simulink Converter/LConn1 -- "Motor & Drive (System Level) "/RConn2
  Simulink-PS Converter/RConn1 -- "Motor & Drive (System Level) "/LConn2
  w/RConn1 -- "Rotational Multibody Interface "/RConn1
  Torque/RConn1 -- "Rotational Multibody Interface "/LConn1

== system UAV_Research_Environment/UAV Plant/UAV Physical [Simscape]/Motor ESC 4 ==
  wCmd : Inport
  Mechanical Rotational Reference1 : fl_lib/Mechanical/Rotational Elements/Mechanical Rotational Reference
  Mechanical Rotational Reference : fl_lib/Mechanical/Rotational Elements/Mechanical Rotational Reference
  "Motor & Drive (System Level) " : ee_lib/Electromechanical/Motor & Drive (System Level)  torque_speed_param=ee.enum.electromech.envelope.torque_power  overtorque_param=ee.enum.electromech.overtorque.no  T_t=[.09, .08, .07, 0] N*m  T_t_intermittent=[.36, .32, .28, 0] N*m  T_t_2D=[.09, .09, .09; .08, .08, .08; .07, .07, .07; 0, 0, 0] N*m  T_t_intermittent_2D=[.36, .36, .36; .32, .32, .32; .28, .28, .28; 0, 0, 0] N*m  w_t=[0, 3750, 7500, 8000] rpm  vdc_t=[6, 12, 24] V  torque_max="P_UAV.drive.max_torque_Nm  N*m"  power_max="P_UAV.drive.max_power_W  W"  torque_max_intermittent=0.4 N*m  power_max_intermittent=120 W  time_overtorque=30 s  time_recover=60 s  Tc="P_UAV.drive.torque_control_time_constant_s  s"  EnableSwitch=false  losses_param=1  eff=P_UAV.drive.efficiency_percent  w_eff="P_UAV.drive.efficiency_speed_rpm  rpm"  T_eff="P_UAV.drive.efficiency_torque_Nm  N*m"  Piron="P_UAV.drive.iron_loss_W  W"  Pbase="P_UAV.drive.fixed_loss_W  W"  w_eff_vec=[-8000, -4000, 0, 4000, 8000] rpm  T_eff_vec=[0, .03, .06, .09] N*m  v_eff_vec=[100, 250, 400] V  losses_mat=[1.49, 1.67, 2.21, 3.1; .42, .69, 1.14, 2.03; .06, .24, .78, 1.68; .42, .69, 1.14, 2.03; 1.49, 1.67, 2.21, 3.1] W  efficiency_mat=[95, 95, 95, 95; 95, 95, 95, 95; 95, 95, 95, 95; 95, 95, 95, 95; 95, 95, 95, 95]  losses_mat_3D=ones(5, 4, 3) W  efficiency_mat_3D=95 * ones(5, 4, 3)  Res=P_UAV.drive.external_supply_resistance_Ohm Ohm  J="P_UAV.drive.rotor_inertia_kgm2  kg*m^2"  lam="P_UAV.drive.rotor_damping_Nm_s_rad  N*m*s/rad"  speed0=P_UAV.drive.initial_speed_rpm rpm  faulted_specify=off  faulted_priority=None  faulted=0  faulted_nominal_specify=off  faulted_nominal_value=1  faulted_nominal_unit=1  isSwitchedOff_specify=off  isSwitchedOff_priority=None  isSwitchedOff=0  isSwitchedOff_nominal_specify=off  isSwitchedOff_nominal_value=1  isSwitchedOff_nominal_unit=1  torqueLimitContinuous_specify=off  torqueLimitContinuous_priority=None  torqueLimitContinuous=0 N*m  torqueLimitContinuous_nominal_specify=off  torqueLimitContinuous_nominal_value=1  torqueLimitContinuous_nominal_unit=N*m  alpha=3.93e-3 1/K  Tmeas=25 degC  Tmeas2=125 degC  losses_mat_T2=[1.49, 1.74, 2.49, 3.74; .42, .67, 1.42, 2.67; .06, .31, 1.06, 2.31; .42, .67, 1.42, 2.67; 1.49, 1.74, 2.49, 3.74] W  efficiency_mat_T2=[95, 95, 95, 95; 95, 95, 95, 95; 95, 95, 95, 95; 95, 95, 95, 95; 95, 95, 95, 95]  losses_mat_3D_T2=ones(5, 4, 3) W  efficiency_mat_3D_T2=95 * ones(5, 4, 3)  thermal_mass=100 J/K  initial_temperature=25 degC
  PS-Simulink Converter : nesl_utility/PS-Simulink Converter  PhysicalDomain=network_engine_domain  SubClassName=ps_output  LeftPortType=input  RightPortType=output  PseudoPeriodic=off  Frequencies=[]  VectorFormat=inherit  Unit=inherit  AffineConversion=off
  "Rotational Multibody Interface " : fl_lib/Mechanical/Multibody Interfaces/Rotational Multibody Interface
  Simulink-PS Converter : nesl_utility/Simulink-PS Converter  PhysicalDomain=network_engine_domain  SubClassName=ps_input  LeftPortType=input  RightPortType=output  PseudoPeriodic=off  Frequencies=[]  NoiseDistribution=none  NoiseParameters=[]  Unit=1  AffineConversion=off  FilteringAndDerivatives=filter  SimscapeFilterOrder=1  InputFilterTimeConstant=0.001  UdotUserProvided=0
  Speed PI Control : Subsystem
  Torque : PMIOPort  Side=Left
  w : PMIOPort  Port=2  Side=Left
  GND : PMIOPort  Port=3  Side=Right
  VCC : PMIOPort  Port=4  Side=Right
  wires:
  PS-Simulink Converter/1 -> Speed PI Control/2(w)
  wCmd/1 -> Speed PI Control/1(wCmd)
  Speed PI Control/1(TorqueCmd) -> Simulink-PS Converter/1
  connections:
  VCC/RConn1 -- "Motor & Drive (System Level) "/LConn1
  "Rotational Multibody Interface "/LConn2 -- Mechanical Rotational Reference/LConn1
  "Rotational Multibody Interface "/RConn2 -- "Motor & Drive (System Level) "/LConn3
  Mechanical Rotational Reference1/LConn1 -- "Motor & Drive (System Level) "/RConn3
  "Motor & Drive (System Level) "/RConn1 -- GND/RConn1
  PS-Simulink Converter/LConn1 -- "Motor & Drive (System Level) "/RConn2
  Simulink-PS Converter/RConn1 -- "Motor & Drive (System Level) "/LConn2
  w/RConn1 -- "Rotational Multibody Interface "/RConn1
  Torque/RConn1 -- "Rotational Multibody Interface "/LConn1

== system UAV_Research_Environment/UAV Plant/UAV Physical [Simscape]/NED Frame ==
  Bus Selector : BusSelector  OutputSignals=Gravity
  Gain : Gain  Gain=|  Multiplication=Matrix(K*u)
      | [1  0  0;
      |  0 -1  0;
      |  0  0 -1]
  Mechanism Configuration : sm_lib/Utilities/Mechanism Configuration  UniformGravity=TimeVarying  GravityVector=P_ENV.gravity.world_vector_m_s2  GravityVectorUnits=m/s^2  LinearizationDelta=0.001  JointModeTransitionNonlinearIterations=2
  Rigid Transform Frame : sm_lib/Frames and Transforms/Rigid Transform  RotationMethod=RotationSequence  FollAlignAxisA=+X  BaseAlignAxisA=+Y  FollAlignAxisB=+Y  BaseAlignAxisB=+Z  RotationStandardAxis=+Z  RotationAngle=0  RotationAngleUnits=deg  RotationArbitraryAxis=[0 0 1]  RotationSequenceAxes=FollowerAxes  RotationSequence=XYZ  RotationSequenceAngles=[180 0 -90]  RotationSequenceAnglesUnits=deg  RotationMatrix=[1 0 0;0 1 0;0 0 1]  Quaternion=[1 0 0 0]  TranslationMethod=None  TranslationCartesianOffset=[0 0 0]  TranslationCartesianOffsetUnits=m  TranslationStandardAxis=+Z  TranslationStandardOffset=0  TranslationStandardOffsetUnits=m  TranslationROffset=0  TranslationROffsetUnits=m  TranslationThetaOffset=0  TranslationThetaOffsetUnits=deg  TranslationZOffset=0  TranslationZOffsetUnits=m
  Simulink-PS Converter : nesl_utility/Simulink-PS Converter  PhysicalDomain=network_engine_domain  SubClassName=ps_input  LeftPortType=input  RightPortType=output  PseudoPeriodic=off  Frequencies=[]  NoiseDistribution=none  NoiseParameters=[]  Unit=m/s^2  AffineConversion=off  FilteringAndDerivatives=provide  SimscapeFilterOrder=1  InputFilterTimeConstant=0.001  UdotUserProvided=0
  Solver Configuration : nesl_utility/Solver Configuration  PhysicalDomain=network_engine_domain  SubClassName=solver  LeftPortType=input  RightPortType=generic  Tones=[]  Harmonics=[]  SimulateNoise=off  Profile=off  UseLocalSampling=off  EnableSwitchedLinearOptims=on  FrequencyDomain=off  UseCCode=off  RelTol=0.001  AbsTol=1e-06  MinStep=1e-09  ToWorkspace=off  RevertToSquareIcSolve=off  NumHomotopyIterations=100  PhasorMode=off  PhasorModeNumHarmonics=1  ConsistencySolver=NEWTON_XTOL_AFTER_FTOL  IndexReductionMethod=DerivativeReplacement  DoDC=off  ResidualTolerance=1e-09  ConsistencyTolSource=GLOBAL  ConsistencyAbsTol=0.001  ConsistencyRelTol=0.001  ConsistencyTolFactor=0.001  UseLocalSolver=off  LocalSolverChoice=NE_BACKWARD_EULER_ADVANCER  ResolveIndetEquations=on  FunctionEvalNumThread=1  LocalSolverSampleTime=0.001  DoFixedCost=off  MaxNonlinIter=3  MaxModeIter=2  ComputeImpulses=off  ImpulseIterations=2  LinearAlgebra=Sparse  LinearAlgebraNumThread=0  EquationFormulation=NE_TIME_EF  DelaysMemoryBudget=1024  AutomaticFiltering=on  FilteringTimeConstant=0.001  PartitionStorageMethod=AS_NEEDED  PartitionMemoryBudget=1024  PartitionMethod=FAST  MultibodyUseLocalSolver=off  MultibodyLocalSolverChoice=ODE1  MultibodyLocalSolverSampleTime=0.001
  World Frame : sm_lib/Frames and Transforms/World Frame
  NED : PMIOPort  Side=Left
  wires:
  [Env] -> Bus Selector/1
  Bus Selector/1 -> Gain/1  "<Gravity>"
  Gain/1 -> Simulink-PS Converter/1
  connections:
  World Frame/RConn1 -- Rigid Transform Frame/LConn1 -- Solver Configuration/RConn1 -- Mechanism Configuration/RConn1
  Rigid Transform Frame/RConn1 -- NED/RConn1
  Simulink-PS Converter/RConn1 -- Mechanism Configuration/LConn1
